simulink model "fbuildv0p3"  (R2024b)
settings: Solver=VariableStepAuto  StartTime=0.0  StopTime=10.0  RelTol=1e-3
model workspace (MAT data in the model file):
  DGain = [16.29965735 16.29965735 15.46224499 15.46224499 15.85491435 21.71073697 22.54158281 11.7271646 11.89023926 12.01707508 12.11854371 12.20156349 12.27074664 12.32928621 12.37946299]
  FBgain = 1
  FFgain = 1
  GR = 14.14
  IGain = [117.4799242 117.4799242 87.54143949 87.54143949 65.86609231 58.19090765 57.39102046 195.6414284 195.4270634 195.2603347 195.1269515 195.0178196 194.9268763 194.8499242 194.7839652]
  Izz = 80
  Kb = 5
  Kd = 2
  Ki = 10
  Kn = 1
  Kp = 0.1
  L = 1.53
  Mz_to_CMD_TV_delta = 1
  NGain = [2.84450804 2.84450804 4.245826716 5.412937893 3.440885499 2 2 14.58729627 14.58729627 14.58729627 14.58729627 14.58729627 14.58729627 14.58729627 14.58729627]
  PGain = [130.03354 130.03354 132.2979663 135.8088906 130.4448578 122.5111241 121.680406 275.8117795 275.6454267 275.5160406 275.4125314 275.3278419 275.2572671 275.1975499 275.1463636]
  R_e = 0.197
  Tmax = 21
  g = 9.81
  h = 0.225
  kappa_desired = 0.2
  mu = 1
  steering_ratio = 1.17517328292
  t = 1.2
  vx_vector = [0 3.21428571429 6.42857142857 9.64285714286 12.8571428571 16.0714285714 19.2857142857 22.5 25.7142857143 28.9285714286 32.1428571429 35.3571428571 38.5714285714 41.7857142857 45]
libraries: slpidlib x2, simulink x1
settings Model: Creator=kara.28  LastModifiedBy=kara.28

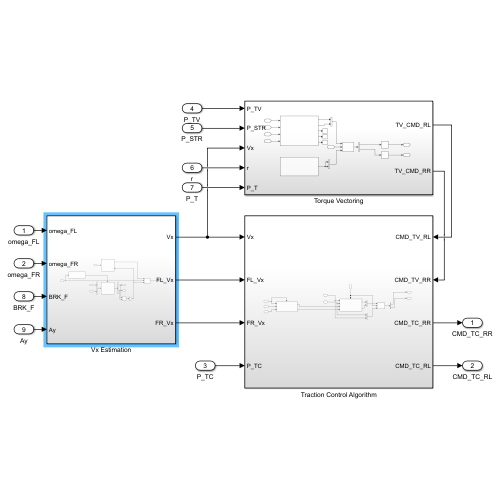
[thumbnail: Simulink's stored preview of the top-level diagram]
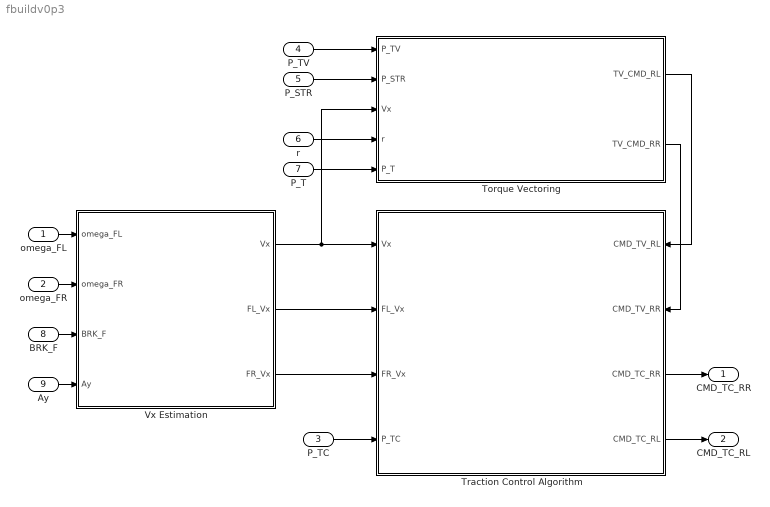
== system fbuildv0p3 ==
  omega_FL : Inport
  omega_FR : Inport  Port=2
  P_TC : Inport  Port=3
  P_TV : Inport  Port=4
  P_STR : Inport  Port=5
  r : Inport  Port=6
  P_T : Inport  Port=7
  BRK_F : Inport  Port=8
  Ay : Inport  Port=9
  Torque Vectoring : Subsystem
  Traction Control Algorithm : Subsystem
      settings: PortSchema="{\"entries\":[{\"content\":{\"sides\":[{\"content\":{\"connectorIds\":[\"In1\",\"In2\",\"In3\",\"In4\"]},\"type\":\"ConnectorPlacement.EquallySpacedRectSide\",\"uuid\":\"6d3224cc-3493-4876-87bf-cb750c54d205\"},{\"content\":{\"connectorIds\":[\"In5\",\"In6\",\"Out1\",\"Out2\"],\"side\":\"RIGHT\"},\"type\":\"ConnectorPlacement.EquallySpacedRectSide\",\"uuid\":\"16bb671c-e18d-4977-8b66-2f7bbb636356\"},{\"content\":{\"side\":\"TOP\"},\"type\":\"ConnectorPlacement.EquallySpacedRectSide\",\"uuid\":\"70c91239-ad82-48f3-8aa3-48d7bdfb7bbb\"}]},\"type\":\"ConnectorPlacement.EquallySpacedConnector\",\"uuid\":\"0f8ba5f7-72f2-430e-8458-63f00911aa7a\"}],\"packageUris\":[\"http://schema.mathworks.com/mf0/Connector/R2020b\"],\"version\":\"1.0\"}"
  Vx Estimation : Subsystem
  CMD_TC_RR : Outport
  CMD_TC_RL : Outport  Port=2
  wires:
  Traction Control Algorithm/2(CMD_TC_RL) -> CMD_TC_RL/1
  Traction Control Algorithm/1(CMD_TC_RR) -> CMD_TC_RR/1
  P_TC/1 -> Traction Control Algorithm/4(P_TC)
  Torque Vectoring/1(TV_CMD_RL) -> Traction Control Algorithm/5(CMD_TV_RL)
  Torque Vectoring/2(TV_CMD_RR) -> Traction Control Algorithm/6(CMD_TV_RR)
  P_TV/1 -> Torque Vectoring/1(P_TV)
  r/1 -> Torque Vectoring/4(r)
  P_T/1 -> Torque Vectoring/5(P_T)
  P_STR/1 -> Torque Vectoring/2(P_STR)
  omega_FL/1 -> Vx Estimation/1(omega_FL)
  omega_FR/1 -> Vx Estimation/2(omega_FR)
  Vx Estimation/2(FL_Vx) -> Traction Control Algorithm/2(FL_Vx)
  Vx Estimation/3(FR_Vx) -> Traction Control Algorithm/3(FR_Vx)
  BRK_F/1 -> Vx Estimation/3(BRK_F)
  Ay/1 -> Vx Estimation/4(Ay)
  Vx Estimation/1(Vx) -> Torque Vectoring/3(Vx), Traction Control Algorithm/1(Vx)

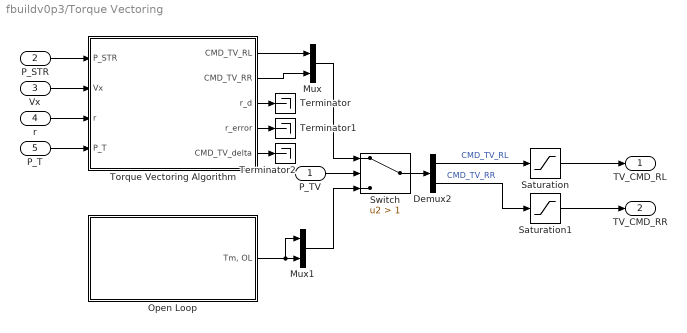
== system fbuildv0p3/Torque Vectoring ==
  P_TV : Inport
  P_STR : Inport  Port=2
  Vx : Inport  Port=3
  r : Inport  Port=4
  P_T : Inport  Port=5
  Demux2 : Demux  Outputs=2
  Mux : Mux  Inputs=2
  Mux1 : Mux  Inputs=2
  Open Loop : Subsystem
  Saturation : Saturate  UpperLimit=Tmax  LowerLimit=0
  Saturation1 : Saturate  UpperLimit=Tmax  LowerLimit=0
  Switch : Switch  Criteria=u2 > Threshold  Threshold=1  SaturateOnIntegerOverflow=off  InputSameDT=off
  Terminator : Terminator
  Terminator1 : Terminator
  Terminator2 : Terminator
  Torque Vectoring Algorithm : Subsystem
  TV_CMD_RL : Outport
  TV_CMD_RR : Outport  Port=2
  wires:
  Demux2/2 -> Saturation1/1  "CMD_TV_RR"
  Mux/1 -> Switch/1
  P_TV/1 -> Switch/2
  Torque Vectoring Algorithm/2(CMD_TV_RR) -> Mux/2
  Demux2/1 -> Saturation/1  "CMD_TV_RL"
  Open Loop/1("Tm, OL") -> Mux1/1, Mux1/2
  Torque Vectoring Algorithm/1(CMD_TV_RL) -> Mux/1
  Mux1/1 -> Switch/3
  Switch/1 -> Demux2/1
  Saturation/1 -> TV_CMD_RL/1
  Saturation1/1 -> TV_CMD_RR/1
  P_STR/1 -> Torque Vectoring Algorithm/1(P_STR)
  Vx/1 -> Torque Vectoring Algorithm/2(Vx)
  r/1 -> Torque Vectoring Algorithm/3(r)
  P_T/1 -> Torque Vectoring Algorithm/4(P_T)
  Torque Vectoring Algorithm/3(r_d) -> Terminator/1
  Torque Vectoring Algorithm/4(r_error) -> Terminator1/1
  Torque Vectoring Algorithm/5(CMD_TV_delta) -> Terminator2/1

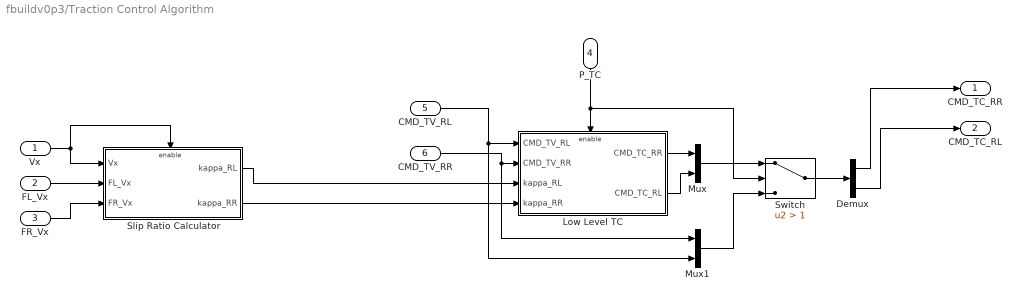
== system fbuildv0p3/Traction Control Algorithm ==
  Vx : Inport
  FL_Vx : Inport  Port=2
  FR_Vx : Inport  Port=3
  P_TC : Inport  Port=4
  CMD_TV_RL : Inport  Port=5
  CMD_TV_RR : Inport  Port=6
  Demux : Demux  Outputs=2
  Low Level TC : Subsystem
  Mux : Mux  Inputs=2
  Mux1 : Mux  Inputs=2
  Slip Ratio Calculator : Subsystem
  Switch : Switch  Criteria=u2 > Threshold  Threshold=1  SaturateOnIntegerOverflow=off  InputSameDT=off
  CMD_TC_RR : Outport
  CMD_TC_RL : Outport  Port=2
  wires:
  Slip Ratio Calculator/2(kappa_RR) -> Low Level TC/4(kappa_RR)
  Slip Ratio Calculator/1(kappa_RL) -> Low Level TC/3(kappa_RL)
  FL_Vx/1 -> Slip Ratio Calculator/2(FL_Vx)
  Vx/1 -> Slip Ratio Calculator/Enable, Slip Ratio Calculator/1(Vx)
  FR_Vx/1 -> Slip Ratio Calculator/3(FR_Vx)
  CMD_TV_RL/1 -> Mux1/2, Low Level TC/1(CMD_TV_RL)
  CMD_TV_RR/1 -> Mux1/1, Low Level TC/2(CMD_TV_RR)
  Low Level TC/1(CMD_TC_RR) -> Mux/1
  Low Level TC/2(CMD_TC_RL) -> Mux/2
  Mux/1 -> Switch/1
  Mux1/1 -> Switch/3
  Switch/1 -> Demux/1
  Demux/1 -> CMD_TC_RR/1
  Demux/2 -> CMD_TC_RL/1
  P_TC/1 -> Switch/2, Low Level TC/Enable

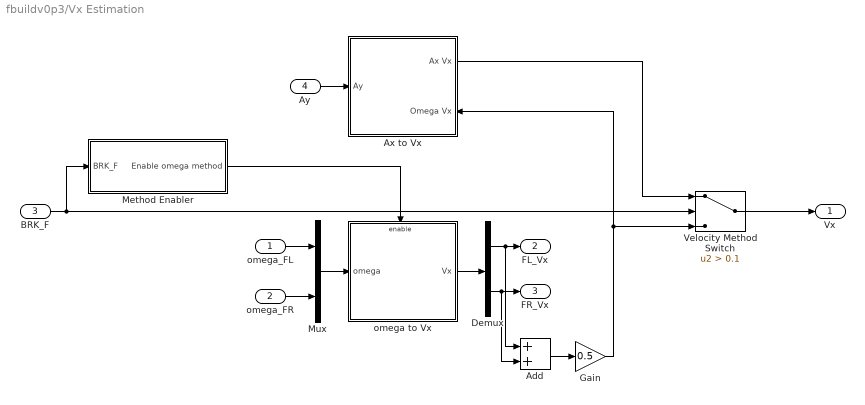
== system fbuildv0p3/Vx Estimation ==
  omega_FL : Inport
  omega_FR : Inport  Port=2
  BRK_F : Inport  Port=3
  Ay : Inport  Port=4
  Add : Sum
  Ax to Vx : Subsystem
      settings: PortSchema="{\"entries\":[{\"content\":{\"sides\":[{\"content\":{\"connectorIds\":[\"In1\"]},\"type\":\"ConnectorPlacement.EquallySpacedRectSide\",\"uuid\":\"79c47d4c-99fc-4629-a356-2be92d656877\"},{\"content\":{\"connectorIds\":[\"Out1\",\"In2\"],\"side\":\"RIGHT\"},\"type\":\"ConnectorPlacement.EquallySpacedRectSide\",\"uuid\":\"a204b3f9-9e82-4b36-9d8a-f01b275c5020\"},{\"content\":{\"side\":\"TOP\"},\"type\":\"ConnectorPlacement.EquallySpacedRectSide\",\"uuid\":\"291354ec-abfe-4550-96ed-63da0986eee3\"}]},\"type\":\"ConnectorPlacement.EquallySpacedConnector\",\"uuid\":\"7bc182f3-54d0-4c5b-b5ad-7c4b2ff36ffe\"}],\"packageUris\":[\"http://schema.mathworks.com/mf0/Connector/R2020b\"],\"version\":\"1.0\"}"
  Demux : Demux  Outputs=2
  Gain : Gain  Gain=0.5
  Method Enabler : Subsystem
  Mux : Mux  Inputs=2
  Velocity Method Switch : Switch  Criteria=u2 > Threshold  Threshold=0.1  SaturateOnIntegerOverflow=off  InputSameDT=off
  omega to Vx : Subsystem
  Vx : Outport
  FL_Vx : Outport  Port=2
  FR_Vx : Outport  Port=3
  wires:
  Mux/1 -> omega to Vx/1(omega)
  omega to Vx/1(Vx) -> Demux/1
  Demux/2 -> Add/2, FR_Vx/1
  omega_FR/1 -> Mux/2
  omega_FL/1 -> Mux/1
  Demux/1 -> Add/1, FL_Vx/1
  BRK_F/1 -> Velocity Method Switch/2, Method Enabler/1(BRK_F)
  Add/1 -> Gain/1
  Gain/1 -> Ax to Vx/2(Omega Vx), Velocity Method Switch/3
  Velocity Method Switch/1 -> Vx/1
  Ay/1 -> Ax to Vx/1(Ay)
  Ax to Vx/1(Ax Vx) -> Velocity Method Switch/1
  Method Enabler/1(Enable omega method) -> omega to Vx/Enable

== system fbuildv0p3/Torque Vectoring/Open Loop ==
  Gain : Gain  Gain=Tmax
  "Tm, OL" : Outport
  wires:
  [throttle] -> Gain/1
  Gain/1 -> "Tm, OL"/1

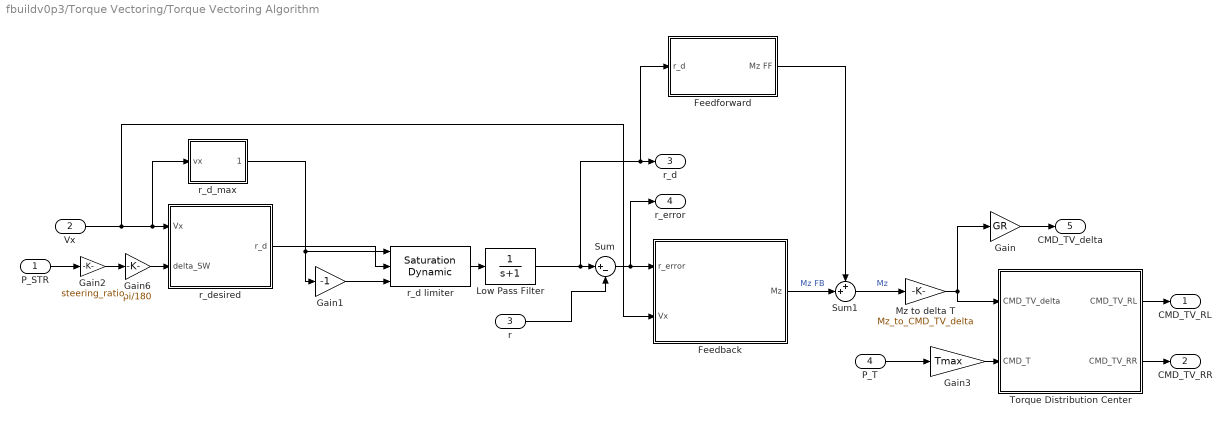
== system fbuildv0p3/Torque Vectoring/Torque Vectoring Algorithm ==
  P_STR : Inport
  Vx : Inport  Port=2
  r : Inport  Port=3
  P_T : Inport  Port=4
  Feedback : Subsystem
  Feedforward : Subsystem
  Gain : Gain  Gain=GR
  Gain1 : Gain  Gain=-1
  Gain2 : Gain  Gain=steering_ratio
  Gain3 : Gain  Gain=Tmax
  Gain6 : Gain  Gain=pi/180
  Low Pass Filter : TransferFcn  Denominator=[1 1]
  Mz to delta T : Gain  Gain=Mz_to_CMD_TV_delta
  Sum : Sum  Inputs=|+-
  Sum1 : Sum  Inputs=++|
  Torque Distribution Center : Subsystem
  r_d limiter : simulink/Discontinuities/Saturation Dynamic  OutMin=[]  OutMax=[]  OutDataTypeStr=Inherit: Same as second input  OutDataType=fixdt(1, 16)  OutScaling=2^-10  RndMeth=Round  DoSatur=off
  r_d_max : Subsystem
  r_desired : Subsystem
  CMD_TV_RL : Outport
  CMD_TV_RR : Outport  Port=2
  r_d : Outport  Port=3
  r_error : Outport  Port=4
  CMD_TV_delta : Outport  Port=5
  wires:
  r_d_max/1(r_d_max) -> r_d limiter/1, Gain1/1
  Sum/1 -> r_error/1, Feedback/1(r_error)
  r_desired/1(r_d) -> r_d limiter/2
  Gain3/1 -> Torque Distribution Center/2(CMD_T)
  r/1 -> Sum/2
  Gain1/1 -> r_d limiter/3
  P_T/1 -> Gain3/1
  Mz to delta T/1 -> Torque Distribution Center/1(CMD_TV_delta), Gain/1
  Gain6/1 -> r_desired/2(delta_SW)
  Vx/1 -> Feedback/2(Vx), r_d_max/1(vx), r_desired/1(Vx)
  Feedback/1(Mz) -> Sum1/2  "Mz FB"
  Sum1/1 -> Mz to delta T/1  "Mz"
  r_d limiter/1 -> Low Pass Filter/1
  Low Pass Filter/1 -> Feedforward/1(r_d), r_d/1, Sum/1
  Feedforward/1(Mz FF) -> Sum1/1
  Torque Distribution Center/1(CMD_TV_RL) -> CMD_TV_RL/1
  Torque Distribution Center/2(CMD_TV_RR) -> CMD_TV_RR/1
  Gain/1 -> CMD_TV_delta/1
  P_STR/1 -> Gain2/1
  Gain2/1 -> Gain6/1

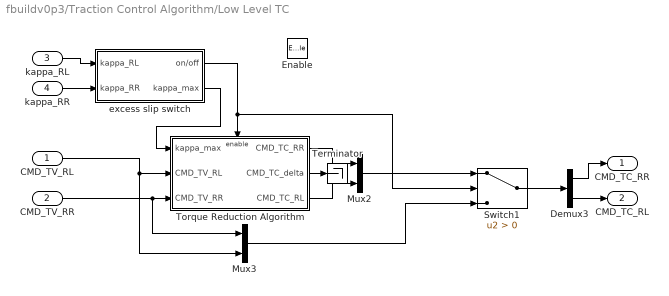
== system fbuildv0p3/Traction Control Algorithm/Low Level TC ==
  CMD_TV_RL : Inport
  CMD_TV_RR : Inport  Port=2
  kappa_RL : Inport  Port=3
  kappa_RR : Inport  Port=4
  Enable : EnablePort
  Demux3 : Demux  Outputs=2
  Mux2 : Mux  Inputs=2
  Mux3 : Mux  Inputs=2
  Switch1 : Switch  Criteria=u2 > Threshold  SaturateOnIntegerOverflow=off  InputSameDT=off
  Terminator : Terminator
  Torque Reduction Algorithm : Subsystem  TreatAsAtomicUnit=on
  excess slip switch : Subsystem
  CMD_TC_RR : Outport
  CMD_TC_RL : Outport  Port=2
  wires:
  Demux3/2 -> CMD_TC_RL/1
  Mux3/1 -> Switch1/3
  CMD_TV_RL/1 -> Mux3/2, Torque Reduction Algorithm/2(CMD_TV_RL)
  Torque Reduction Algorithm/2(CMD_TC_delta) -> Terminator/1
  CMD_TV_RR/1 -> Mux3/1, Torque Reduction Algorithm/3(CMD_TV_RR)
  Torque Reduction Algorithm/1(CMD_TC_RR) -> Mux2/1
  excess slip switch/1(on/off) -> Switch1/2, Torque Reduction Algorithm/Enable
  Mux2/1 -> Switch1/1
  Torque Reduction Algorithm/3(CMD_TC_RL) -> Mux2/2
  Switch1/1 -> Demux3/1
  Demux3/1 -> CMD_TC_RR/1
  excess slip switch/2(kappa_max) -> Torque Reduction Algorithm/1(kappa_max)
  kappa_RL/1 -> excess slip switch/1(kappa_RL)
  kappa_RR/1 -> excess slip switch/2(kappa_RR)

== system fbuildv0p3/Traction Control Algorithm/Slip Ratio Calculator ==
  Vx : Inport
  FL_Vx : Inport  Port=2
  FR_Vx : Inport  Port=3
  Enable : EnablePort
  Divide : Product  Inputs=*/
  Divide1 : Product  Inputs=*/
  Subtract : Sum  Inputs=+-
  Subtract1 : Sum  Inputs=+-
  kappa_RL : Outport
  kappa_RR : Outport  Port=2
  wires:
  Subtract/1 -> Divide/1
  Vx/1 -> Subtract1/1, Divide/2, Divide1/2, Subtract/1
  Divide/1 -> kappa_RL/1
  Divide1/1 -> kappa_RR/1
  Subtract1/1 -> Divide1/1
  FL_Vx/1 -> Subtract/2
  FR_Vx/1 -> Subtract1/2

== system fbuildv0p3/Vx Estimation/Ax to Vx ==
  Ay : Inport
  Omega Vx : Inport  Port=2
  Integrator : Integrator
  Plus : Sum
  Ax Vx : Outport
  wires:
  Ay/1 -> Integrator/1
  Integrator/1 -> Plus/2
  Omega Vx/1 -> Plus/1
  Plus/1 -> Ax Vx/1

== system fbuildv0p3/Vx Estimation/Method Enabler ==
  BRK_F : Inport
  Constant : Constant  Value=0
  Constant1 : Constant
  Switch : Switch  Criteria=u2 > Threshold  Threshold=0.1  SaturateOnIntegerOverflow=off  InputSameDT=off
  Enable omega method : Outport
  wires:
  Constant1/1 -> Switch/3
  Constant/1 -> Switch/1
  Switch/1 -> Enable omega method/1
  BRK_F/1 -> Switch/2

== system fbuildv0p3/Vx Estimation/omega to Vx ==
  omega : Inport
  Enable : EnablePort
  Gain : Gain  Gain=R_e
  Vx : Outport
  wires:
  omega/1 -> Gain/1
  Gain/1 -> Vx/1

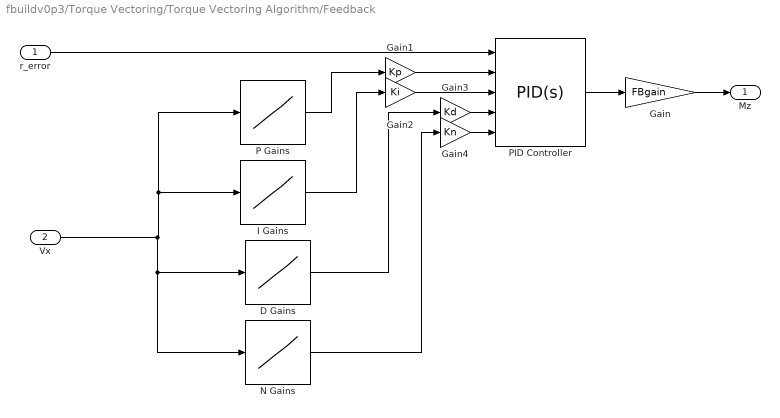
== system fbuildv0p3/Torque Vectoring/Torque Vectoring Algorithm/Feedback ==
  r_error : Inport
  Vx : Inport  Port=2
  D Gains : Lookup_n-D  NumberOfTableDimensions=1  LookupTableObject=''  BreakpointsForDimension1=vx_vector  BreakpointsForDimension1FirstPoint=10  BreakpointsForDimension2FirstPoint=10  BreakpointsForDimension1Spacing=12  BreakpointsForDimension2Spacing=12  IndexSearchMethod=Evenly spaced points  Table=DGain  RemoveProtectionInput=on  InternalRulePriority=Speed  RndMeth=Simplest
  Gain : Gain  Gain=FBgain
  Gain1 : Gain  Gain=Kp
  Gain2 : Gain  Gain=Ki
  Gain3 : Gain  Gain=Kd
  Gain4 : Gain  Gain=Kn
  I Gains : Lookup_n-D  NumberOfTableDimensions=1  LookupTableObject=''  BreakpointsForDimension1=vx_vector  BreakpointsForDimension1FirstPoint=10  BreakpointsForDimension2FirstPoint=10  BreakpointsForDimension1Spacing=12  BreakpointsForDimension2Spacing=12  IndexSearchMethod=Evenly spaced points  Table=IGain  RemoveProtectionInput=on  InternalRulePriority=Speed  RndMeth=Simplest
  N Gains : Lookup_n-D  NumberOfTableDimensions=1  LookupTableObject=''  BreakpointsForDimension1=vx_vector  BreakpointsForDimension1FirstPoint=10  BreakpointsForDimension2FirstPoint=10  BreakpointsForDimension1Spacing=12  BreakpointsForDimension2Spacing=12  IndexSearchMethod=Evenly spaced points  Table=NGain  RemoveProtectionInput=on  InternalRulePriority=Speed  RndMeth=Simplest
  P Gains : Lookup_n-D  NumberOfTableDimensions=1  LookupTableObject=''  BreakpointsForDimension1=vx_vector  BreakpointsForDimension1FirstPoint=10  BreakpointsForDimension2FirstPoint=10  BreakpointsForDimension1Spacing=12  BreakpointsForDimension2Spacing=12  IndexSearchMethod=Evenly spaced points  Table=PGain  RemoveProtectionInput=on  InternalRulePriority=Speed  RndMeth=Simplest
  PID Controller : slpidlib/PID Controller  Controller=PID  Form=Parallel  TimeDomain=Continuous-time  UseExternalTs=off  SampleTime=-1  IntegratorMethod=Forward Euler  FilterMethod=Forward Euler  ControllerParametersSource=external  P=122.511124072632  I=58.1909076470783  UseKiTs=off  D=21.7107369694367  UseExternalDerivativeSource=off  N=2  UseFilter=on  TunerSelectOption=Transfer Function Based (PID Tuner App)  InitialConditionSource=internal  InitialConditionForIntegrator=0  InitialConditionForFilter=0  DifferentiatorICPrevScaledInput=0  ExternalReset=none  TrackingMode=off  Kt=1  LimitOutput=on  SatLimitsSource=internal  UpperSaturationLimit=10  LowerSaturationLimit=-10  LinearizeAsGain=on  AntiWindupMode=back-calculation  Kb=Kb  LimitIntegrator=off  UpperIntegratorSaturationLimit=inf  LowerIntegratorSaturationLimit=-inf  POutMin=[]  POutMax=[]  IOutMin=[]  IOutMax=[]  DOutMin=[]  DOutMax=[]  NOutMin=[]  NOutMax=[]  SumOutMin=[]  SumOutMax=[]  SaturationOutMin=[]  SaturationOutMax=[]  PParamMin=[]  PParamMax=[]  IParamMin=[]  IParamMax=[]  DParamMin=[]  DParamMax=[]  NParamMin=[]  NParamMax=[]  KbParamMin=[]  KbParamMax=[]  KtParamMin=[]  KtParamMax=[]  KbOutMin=[]  KbOutMax=[]  KtOutMin=[]  KtOutMax=[]  IntegratorOutMin=[]  IntegratorOutMax=[]  FilterOutMin=[]  FilterOutMax=[]  SumI1OutMin=[]  SumI1OutMax=[]  SumI2OutMin=[]  SumI2OutMax=[]  SumI3OutMin=[]  SumI3OutMax=[]  SumI4OutMin=[]  SumI4OutMax=[]  SumDOutMin=[]  SumDOutMax=[]  DifferentiatorOutMin=[]  DifferentiatorOutMax=[]  FilterDiffOutCoefMin=[]  FilterDiffOutCoefMax=[]  ReciprocalOutMin=[]  ReciprocalOutMax=[]  SumDenOutMin=[]  SumDenOutMax=[]  SumNumOutMin=[]  SumNumOutMax=[]  DivideOutMin=[]  DivideOutMax=[]  UdiffTsProdOutMin=[]  UdiffTsProdOutMax=[]  NTsProdOutMin=[]  NTsProdOutMax=[]  UintegralTsProdOutMin=[]  UintegralTsProdOutMax=[]  UngainTsProdOutMin=[]  UngainTsProdOutMax=[]  ClampingZeroOutDataTypeStr=Inherit: Inherit via back propagation  ClampingZeroOutMin=[]  ClampingZeroOutMax=[]  FilterDenConstantOutDataTypeStr=Inherit: Inherit via back propagation  FilterDenConstantOutMin=[]  FilterDenConstantOutMax=[]  PCopyOutDataTypeStr=Inherit: Inherit via back propagation  PCopyOutMin=[]  PCopyOutMax=[]  NCopyOutDataTypeStr=Inherit: Inherit via back propagation  NCopyOutMin=[]  NCopyOutMax=[]  IntegratorContinuousStateAttributes=''  IntegratorStateMustResolveToSignalObject=off  IntegratorRTWStateStorageClass=Auto  FilterContinuousStateAttributes=''  FilterStateMustResolveToSignalObject=off  FilterRTWStateStorageClass=Auto  ParallelPVariant=ExternalParameters  IdealPVariant=Disabled  IVariant=ExternalParameters  DVariant=ExternalParameters  IntegratorVariant=Continuous  SatVariant=Enabled  AWVariant=BackCalculation  PCopyVariant=Disabled  TRVariant=Disabled  FdbkBlocksVariant=Forward  IdealPFdbkVariant=Disabled  SatFdbkVariant=Disabled  DerivativeFilterVariant=ContFilter  NVariant=ExternalParameters  NCopyVariant=Disabled  FilterICVariant=InternalICsFilter  IntegratorICVariant=InternalICs  ExternalResetVariant=Disabled  TRSumVariant=Passthrough  SumFdbkVariant=Disabled  SumVariant=Sum_PID  TsampFilterVariant=InternalTs  TsampNgainVariant=Passthrough  TsampIntegralVariant=Disabled_SignalSpec  ExternalSaturationOutDataTypeStr=Inherit: Same as second input  DerivativeSourceVariant=ErrorSignal  PreIntVariant=InternalPreInt
  Mz : Outport
  wires:
  r_error/1 -> PID Controller/1
  Vx/1 -> N Gains/1, D Gains/1, I Gains/1, P Gains/1
  I Gains/1 -> Gain2/1
  N Gains/1 -> Gain4/1
  PID Controller/1 -> Gain/1
  Gain/1 -> Mz/1
  P Gains/1 -> Gain1/1
  D Gains/1 -> Gain3/1
  Gain1/1 -> PID Controller/2
  Gain2/1 -> PID Controller/3
  Gain3/1 -> PID Controller/4
  Gain4/1 -> PID Controller/5

== system fbuildv0p3/Torque Vectoring/Torque Vectoring Algorithm/Feedforward ==
  r_d : Inport
  Gain : Gain  Gain=Izz
  Gain2 : Gain  Gain=FFgain
  Mz FF : Outport
  wires:
  r_d/1 -> Gain/1
  Gain/1 -> Gain2/1
  Gain2/1 -> Mz FF/1  "Mz FF"

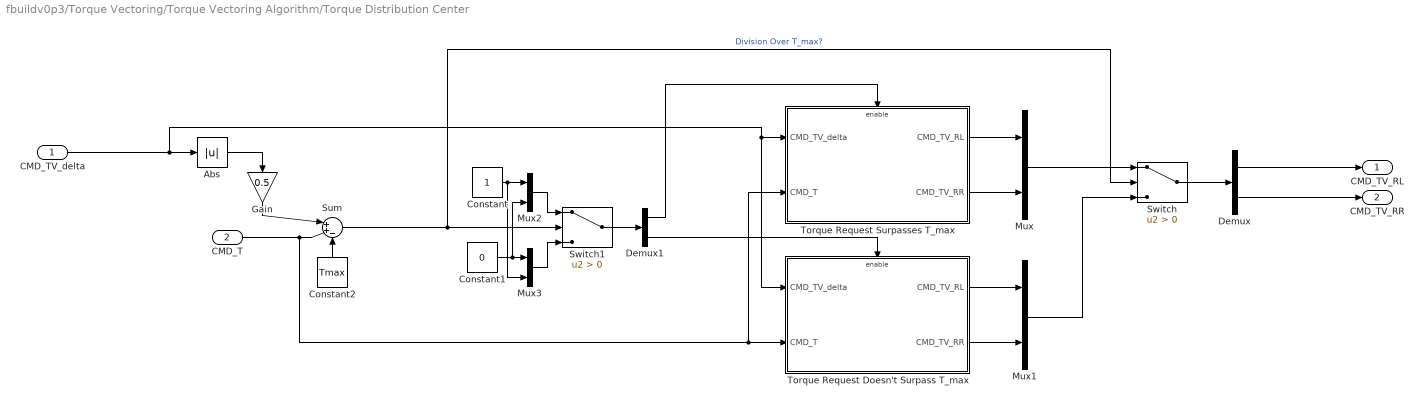
== system fbuildv0p3/Torque Vectoring/Torque Vectoring Algorithm/Torque Distribution Center ==
  CMD_TV_delta : Inport
  CMD_T : Inport  Port=2
  Abs : Abs  SaturateOnIntegerOverflow=off
  Constant : Constant
  Constant1 : Constant  Value=0
  Constant2 : Constant  Value=Tmax
  Demux : Demux  Outputs=2
  Demux1 : Demux  Outputs=2
  Gain : Gain  Gain=0.5
  Mux{,1..3} (4 alike) : Mux  Inputs=2
  Sum : Sum  Inputs=|++-
  Switch : Switch  Criteria=u2 > Threshold  SaturateOnIntegerOverflow=off  InputSameDT=off
  Switch1 : Switch  Criteria=u2 > Threshold  SaturateOnIntegerOverflow=off  InputSameDT=off
  Torque Request Doesn't Surpass T_max : Subsystem  TreatAsAtomicUnit=on
  Torque Request Surpasses T_max : Subsystem  TreatAsAtomicUnit=on
  CMD_TV_RL : Outport
  CMD_TV_RR : Outport  Port=2
  wires:
  Sum/1 -> Switch1/2, Switch/2  "Division Over T_max?"
  Gain/1 -> Sum/1
  Abs/1 -> Gain/1
  Torque Request Surpasses T_max/1(CMD_TV_RL) -> Mux/1
  Torque Request Surpasses T_max/2(CMD_TV_RR) -> Mux/2
  Torque Request Doesn't Surpass T_max/1(CMD_TV_RL) -> Mux1/1
  Torque Request Doesn't Surpass T_max/2(CMD_TV_RR) -> Mux1/2
  Mux/1 -> Switch/1
  Mux1/1 -> Switch/3
  Switch/1 -> Demux/1
  CMD_T/1 -> Torque Request Surpasses T_max/2(CMD_T), Torque Request Doesn't Surpass T_max/2(CMD_T), Sum/2
  Mux2/1 -> Switch1/1
  Mux3/1 -> Switch1/3
  Switch1/1 -> Demux1/1
  Demux1/1 -> Torque Request Surpasses T_max/Enable
  Demux1/2 -> Torque Request Doesn't Surpass T_max/Enable
  Constant/1 -> Mux2/1, Mux3/2
  Constant1/1 -> Mux2/2, Mux3/1
  CMD_TV_delta/1 -> Torque Request Doesn't Surpass T_max/1(CMD_TV_delta), Torque Request Surpasses T_max/1(CMD_TV_delta), Abs/1
  Demux/1 -> CMD_TV_RL/1
  Demux/2 -> CMD_TV_RR/1
  Constant2/1 -> Sum/3

== system fbuildv0p3/Torque Vectoring/Torque Vectoring Algorithm/r_d_max ==
  vx : Inport
  Constant : Constant  Value=0.85*mu*g/(1+(h/t))
  Divide : Product  Inputs=*/
  Saturation : Saturate  UpperLimit=1000000  LowerLimit=0.01
  r_d_max : Outport
  wires:
  Constant/1 -> Divide/1
  vx/1 -> Saturation/1
  Saturation/1 -> Divide/2
  Divide/1 -> r_d_max/1

== system fbuildv0p3/Torque Vectoring/Torque Vectoring Algorithm/r_desired ==
  Vx : Inport
  delta_SW : Inport  Port=2
  Gain : Gain  Gain=1/L
  Product : Product
  Tan : Trigonometry  Operator=tan
  r_d : Outport
  wires:
  delta_SW/1 -> Tan/1
  Vx/1 -> Product/1
  Tan/1 -> Product/2
  Product/1 -> Gain/1
  Gain/1 -> r_d/1

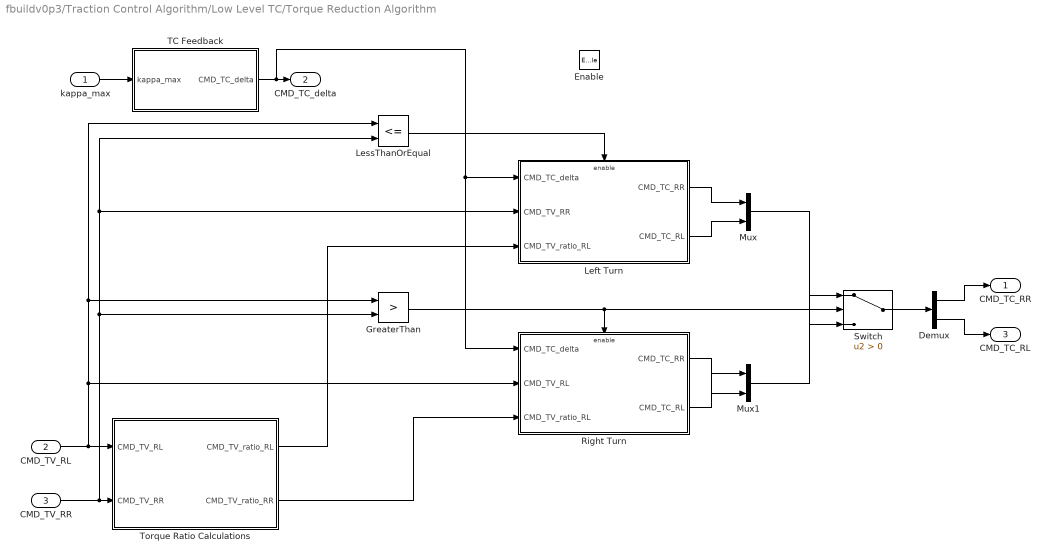
== system fbuildv0p3/Traction Control Algorithm/Low Level TC/Torque Reduction Algorithm ==
  kappa_max : Inport
  CMD_TV_RL : Inport  Port=2
  CMD_TV_RR : Inport  Port=3
  Enable : EnablePort
  Demux : Demux  Outputs=2
  GreaterThan : RelationalOperator  Operator=>  OutDataTypeStr=boolean  RndMeth=Simplest  InputSameDT=off
  Left Turn : Subsystem  TreatAsAtomicUnit=on
  LessThanOrEqual : RelationalOperator  Operator=<=  OutDataTypeStr=boolean  RndMeth=Simplest  InputSameDT=off
  Mux : Mux  Inputs=2
  Mux1 : Mux  Inputs=2
  Right Turn : Subsystem  TreatAsAtomicUnit=on
  Switch : Switch  Criteria=u2 > Threshold  SaturateOnIntegerOverflow=off  InputSameDT=off
  TC Feedback : Subsystem
  Torque Ratio Calculations : Subsystem
  CMD_TC_RR : Outport
  CMD_TC_delta : Outport  Port=2
  CMD_TC_RL : Outport  Port=3
  wires:
  CMD_TV_RL/1 -> GreaterThan/1, LessThanOrEqual/1, Right Turn/2(CMD_TV_RL), Torque Ratio Calculations/1(CMD_TV_RL)
  CMD_TV_RR/1 -> GreaterThan/2, LessThanOrEqual/2, Left Turn/2(CMD_TV_RR), Torque Ratio Calculations/2(CMD_TV_RR)
  LessThanOrEqual/1 -> Left Turn/Enable
  GreaterThan/1 -> Switch/2, Right Turn/Enable
  kappa_max/1 -> TC Feedback/1(kappa_max)
  TC Feedback/1(CMD_TC_delta) -> Right Turn/1(CMD_TC_delta), Left Turn/1(CMD_TC_delta), CMD_TC_delta/1
  Torque Ratio Calculations/1(CMD_TV_ratio_RL) -> Left Turn/3(CMD_TV_ratio_RL)
  Torque Ratio Calculations/2(CMD_TV_ratio_RR) -> Right Turn/3(CMD_TV_ratio_RL)
  Left Turn/1(CMD_TC_RR) -> Mux/1
  Left Turn/2(CMD_TC_RL) -> Mux/2
  Right Turn/2(CMD_TC_RL) -> Mux1/1
  Right Turn/1(CMD_TC_RR) -> Mux1/2
  Mux/1 -> Switch/3
  Mux1/1 -> Switch/1
  Switch/1 -> Demux/1
  Demux/1 -> CMD_TC_RR/1
  Demux/2 -> CMD_TC_RL/1

== system fbuildv0p3/Traction Control Algorithm/Low Level TC/excess slip switch ==
  kappa_RL : Inport
  kappa_RR : Inport  Port=2
  Constant : Constant
  Constant2 : Constant  Value=0
  Max : MinMax  Function=max  Inputs=2
  Switch1 : Switch  Criteria=u2 > Threshold  Threshold=kappa_desired  SaturateOnIntegerOverflow=off  InputSameDT=off
  on/off : Outport
  kappa_max : Outport  Port=2
  wires:
  kappa_RL/1 -> Max/1
  kappa_RR/1 -> Max/2
  Switch1/1 -> on/off/1
  Max/1 -> kappa_max/1, Switch1/2
  Constant2/1 -> Switch1/3
  Constant/1 -> Switch1/1

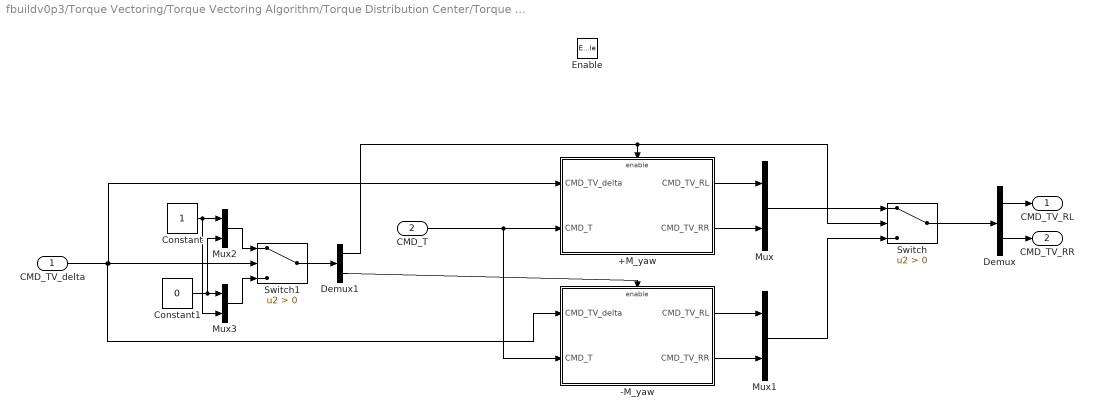
== system fbuildv0p3/Torque Vectoring/Torque Vectoring Algorithm/Torque Distribution Center/Torque Request Doesn't Surpass T_max ==
  CMD_TV_delta : Inport
  CMD_T : Inport  Port=2
  Enable : EnablePort  StatesWhenEnabling=reset
  +M_yaw : Subsystem  TreatAsAtomicUnit=on
  -M_yaw : Subsystem  TreatAsAtomicUnit=on
  Constant : Constant
  Constant1 : Constant  Value=0
  Demux : Demux  Outputs=2
  Demux1 : Demux  Outputs=2
  Mux{,1..3} (4 alike) : Mux  Inputs=2
  Switch : Switch  Criteria=u2 > Threshold  SaturateOnIntegerOverflow=off  InputSameDT=off
  Switch1 : Switch  Criteria=u2 > Threshold  SaturateOnIntegerOverflow=off  InputSameDT=off
  CMD_TV_RL : Outport
  CMD_TV_RR : Outport  Port=2
  wires:
  +M_yaw/1(CMD_TV_RL) -> Mux/1
  +M_yaw/2(CMD_TV_RR) -> Mux/2
  -M_yaw/1(CMD_TV_RL) -> Mux1/1
  -M_yaw/2(CMD_TV_RR) -> Mux1/2
  Mux/1 -> Switch/1
  Mux1/1 -> Switch/3
  CMD_T/1 -> -M_yaw/2(CMD_T), +M_yaw/2(CMD_T)
  Switch/1 -> Demux/1
  Demux/1 -> CMD_TV_RL/1
  Demux/2 -> CMD_TV_RR/1
  Mux2/1 -> Switch1/1
  Demux1/1 -> Switch/2, +M_yaw/Enable
  Demux1/2 -> -M_yaw/Enable
  Mux3/1 -> Switch1/3
  Switch1/1 -> Demux1/1
  Constant1/1 -> Mux2/2, Mux3/1
  Constant/1 -> Mux2/1, Mux3/2
  CMD_TV_delta/1 -> Switch1/2, +M_yaw/1(CMD_TV_delta), -M_yaw/1(CMD_TV_delta)

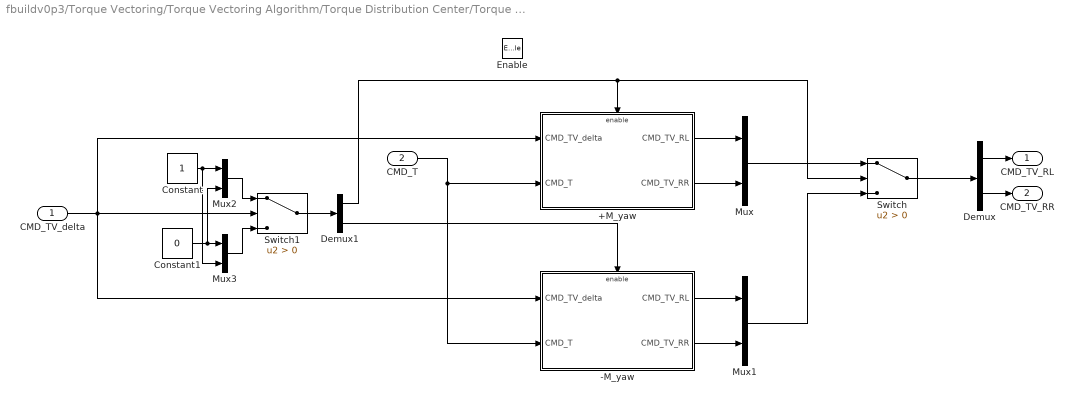
== system fbuildv0p3/Torque Vectoring/Torque Vectoring Algorithm/Torque Distribution Center/Torque Request Surpasses T_max ==
  CMD_TV_delta : Inport
  CMD_T : Inport  Port=2
  Enable : EnablePort  StatesWhenEnabling=reset
  +M_yaw : Subsystem  TreatAsAtomicUnit=on
  -M_yaw : Subsystem  TreatAsAtomicUnit=on
  Constant : Constant
  Constant1 : Constant  Value=0
  Demux : Demux  Outputs=2
  Demux1 : Demux  Outputs=2
  Mux{,1..3} (4 alike) : Mux  Inputs=2
  Switch : Switch  Criteria=u2 > Threshold  SaturateOnIntegerOverflow=off  InputSameDT=off
  Switch1 : Switch  Criteria=u2 > Threshold  SaturateOnIntegerOverflow=off  InputSameDT=off
  CMD_TV_RL : Outport
  CMD_TV_RR : Outport  Port=2
  wires:
  Mux/1 -> Switch/1
  Mux1/1 -> Switch/3
  CMD_T/1 -> -M_yaw/2(CMD_T), +M_yaw/2(CMD_T)
  Demux/2 -> CMD_TV_RR/1
  Demux/1 -> CMD_TV_RL/1
  +M_yaw/2(CMD_TV_RR) -> Mux/2
  +M_yaw/1(CMD_TV_RL) -> Mux/1
  -M_yaw/2(CMD_TV_RR) -> Mux1/2
  Switch/1 -> Demux/1
  -M_yaw/1(CMD_TV_RL) -> Mux1/1
  Mux2/1 -> Switch1/1
  Demux1/1 -> +M_yaw/Enable, Switch/2
  Demux1/2 -> -M_yaw/Enable
  Mux3/1 -> Switch1/3
  Switch1/1 -> Demux1/1
  Constant1/1 -> Mux2/2, Mux3/1
  Constant/1 -> Mux2/1, Mux3/2
  CMD_TV_delta/1 -> Switch1/2, -M_yaw/1(CMD_TV_delta), +M_yaw/1(CMD_TV_delta)

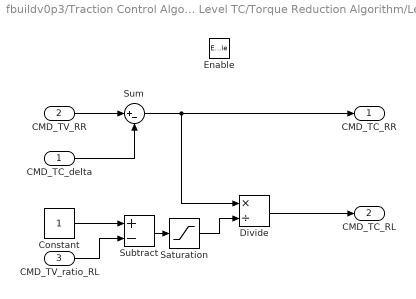
== system fbuildv0p3/Traction Control Algorithm/Low Level TC/Torque Reduction Algorithm/Left Turn ==
  CMD_TC_delta : Inport
  CMD_TV_RR : Inport  Port=2
  CMD_TV_ratio_RL : Inport  Port=3
  Enable : EnablePort
  Constant : Constant
  Divide : Product  Inputs=*/
  Saturation : Saturate  UpperLimit=inf  LowerLimit=0.001
  Subtract : Sum  Inputs=+-
  Sum : Sum  Inputs=|+-
  CMD_TC_RR : Outport
  CMD_TC_RL : Outport  Port=2
  wires:
  CMD_TV_RR/1 -> Sum/1
  CMD_TC_delta/1 -> Sum/2
  Constant/1 -> Subtract/1
  CMD_TV_ratio_RL/1 -> Subtract/2
  Sum/1 -> Divide/1, CMD_TC_RR/1
  Subtract/1 -> Saturation/1
  Saturation/1 -> Divide/2
  Divide/1 -> CMD_TC_RL/1

== system fbuildv0p3/Traction Control Algorithm/Low Level TC/Torque Reduction Algorithm/Right Turn ==
  CMD_TC_delta : Inport
  CMD_TV_RL : Inport  Port=2
  CMD_TV_ratio_RL : Inport  Port=3
  Enable : EnablePort
  Constant : Constant
  Divide : Product  Inputs=*/
  Saturation : Saturate  UpperLimit=inf  LowerLimit=0.001
  Subtract : Sum  Inputs=+-
  Sum : Sum  Inputs=|+-
  CMD_TC_RR : Outport
  CMD_TC_RL : Outport  Port=2
  wires:
  Sum/1 -> Divide/1, CMD_TC_RL/1
  CMD_TC_delta/1 -> Sum/2
  CMD_TV_ratio_RL/1 -> Subtract/2
  Saturation/1 -> Divide/2
  Constant/1 -> Subtract/1
  Subtract/1 -> Saturation/1
  Divide/1 -> CMD_TC_RR/1
  CMD_TV_RL/1 -> Sum/1

== system fbuildv0p3/Traction Control Algorithm/Low Level TC/Torque Reduction Algorithm/TC Feedback ==
  kappa_max : Inport
  Constant : Constant  Value=kappa_desired
  PID Controller : slpidlib/PID Controller  Controller=PID  Form=Parallel  TimeDomain=Continuous-time  UseExternalTs=off  SampleTime=-1  IntegratorMethod=Forward Euler  FilterMethod=Forward Euler  ControllerParametersSource=internal  P=1  I=1  UseKiTs=off  D=0  UseExternalDerivativeSource=off  N=100  UseFilter=on  TunerSelectOption=Transfer Function Based (PID Tuner App)  InitialConditionSource=internal  InitialConditionForIntegrator=0  InitialConditionForFilter=0  DifferentiatorICPrevScaledInput=0  ExternalReset=none  TrackingMode=off  Kt=1  LimitOutput=off  SatLimitsSource=internal  UpperSaturationLimit=inf  LowerSaturationLimit=-inf  LinearizeAsGain=on  AntiWindupMode=none  Kb=1  LimitIntegrator=off  UpperIntegratorSaturationLimit=inf  LowerIntegratorSaturationLimit=-inf  POutMin=[]  POutMax=[]  IOutMin=[]  IOutMax=[]  DOutMin=[]  DOutMax=[]  NOutMin=[]  NOutMax=[]  SumOutMin=[]  SumOutMax=[]  SaturationOutMin=[]  SaturationOutMax=[]  PParamMin=[]  PParamMax=[]  IParamMin=[]  IParamMax=[]  DParamMin=[]  DParamMax=[]  NParamMin=[]  NParamMax=[]  KbParamMin=[]  KbParamMax=[]  KtParamMin=[]  KtParamMax=[]  KbOutMin=[]  KbOutMax=[]  KtOutMin=[]  KtOutMax=[]  IntegratorOutMin=[]  IntegratorOutMax=[]  FilterOutMin=[]  FilterOutMax=[]  SumI1OutMin=[]  SumI1OutMax=[]  SumI2OutMin=[]  SumI2OutMax=[]  SumI3OutMin=[]  SumI3OutMax=[]  SumI4OutMin=[]  SumI4OutMax=[]  SumDOutMin=[]  SumDOutMax=[]  DifferentiatorOutMin=[]  DifferentiatorOutMax=[]  FilterDiffOutCoefMin=[]  FilterDiffOutCoefMax=[]  ReciprocalOutMin=[]  ReciprocalOutMax=[]  SumDenOutMin=[]  SumDenOutMax=[]  SumNumOutMin=[]  SumNumOutMax=[]  DivideOutMin=[]  DivideOutMax=[]  UdiffTsProdOutMin=[]  UdiffTsProdOutMax=[]  NTsProdOutMin=[]  NTsProdOutMax=[]  UintegralTsProdOutMin=[]  UintegralTsProdOutMax=[]  UngainTsProdOutMin=[]  UngainTsProdOutMax=[]  ClampingZeroOutDataTypeStr=Inherit: Inherit via back propagation  ClampingZeroOutMin=[]  ClampingZeroOutMax=[]  FilterDenConstantOutDataTypeStr=Inherit: Inherit via back propagation  FilterDenConstantOutMin=[]  FilterDenConstantOutMax=[]  PCopyOutDataTypeStr=Inherit: Inherit via back propagation  PCopyOutMin=[]  PCopyOutMax=[]  NCopyOutDataTypeStr=Inherit: Inherit via back propagation  NCopyOutMin=[]  NCopyOutMax=[]  IntegratorContinuousStateAttributes=''  IntegratorStateMustResolveToSignalObject=off  IntegratorRTWStateStorageClass=Auto  FilterContinuousStateAttributes=''  FilterStateMustResolveToSignalObject=off  FilterRTWStateStorageClass=Auto  ParallelPVariant=InternalParameters  IdealPVariant=Disabled  IVariant=InternalParameters  DVariant=InternalParameters  IntegratorVariant=Continuous  SatVariant=Disabled  AWVariant=Passthrough  PCopyVariant=Disabled  TRVariant=Disabled  FdbkBlocksVariant=Forward  IdealPFdbkVariant=Disabled  SatFdbkVariant=Disabled  DerivativeFilterVariant=ContFilter  NVariant=InternalParameters  NCopyVariant=Disabled  FilterICVariant=InternalICsFilter  IntegratorICVariant=InternalICs  ExternalResetVariant=Disabled  TRSumVariant=Passthrough  SumFdbkVariant=Disabled  SumVariant=Sum_PID  TsampFilterVariant=InternalTs  TsampNgainVariant=Passthrough  TsampIntegralVariant=Disabled_SignalSpec  ExternalSaturationOutDataTypeStr=Inherit: Same as second input  DerivativeSourceVariant=ErrorSignal  PreIntVariant=InternalPreInt
  Saturation : Saturate  UpperLimit=Tmax  LowerLimit=0
  Sum : Sum  Inputs=|+-
  CMD_TC_delta : Outport
  wires:
  Constant/1 -> Sum/1
  Sum/1 -> PID Controller/1
  PID Controller/1 -> Saturation/1
  kappa_max/1 -> Sum/2
  Saturation/1 -> CMD_TC_delta/1

== system fbuildv0p3/Traction Control Algorithm/Low Level TC/Torque Reduction Algorithm/Torque Ratio Calculations ==
  CMD_TV_RL : Inport
  CMD_TV_RR : Inport  Port=2
  Divide : Product  Inputs=*/
  Divide1 : Product  Inputs=*/
  Saturation : Saturate  UpperLimit=inf  LowerLimit=0.001
  Sum : Sum  Inputs=|++
  CMD_TV_ratio_RL : Outport
  CMD_TV_ratio_RR : Outport  Port=2
  wires:
  CMD_TV_RL/1 -> Divide/1, Sum/1
  CMD_TV_RR/1 -> Sum/2, Divide1/1
  Sum/1 -> Saturation/1
  Saturation/1 -> Divide1/2, Divide/2
  Divide/1 -> CMD_TV_ratio_RL/1
  Divide1/1 -> CMD_TV_ratio_RR/1

== system fbuildv0p3/Torque Vectoring/Torque Vectoring Algorithm/Torque Distribution Center/Torque Request Doesn't Surpass T_max/+M_yaw ==
  CMD_TV_delta : Inport
  CMD_T : Inport  Port=2
  Enable : EnablePort  StatesWhenEnabling=reset
  Abs : Abs  SaturateOnIntegerOverflow=off
  Add : Sum
  Gain : Gain  Gain=0.5
  Subtract : Sum  Inputs=+-
  CMD_TV_RL : Outport
  CMD_TV_RR : Outport  Port=2
  wires:
  CMD_TV_delta/1 -> Abs/1
  Abs/1 -> Gain/1
  Gain/1 -> Add/2, Subtract/2
  CMD_T/1 -> Subtract/1, Add/1
  Subtract/1 -> CMD_TV_RL/1
  Add/1 -> CMD_TV_RR/1

== system fbuildv0p3/Torque Vectoring/Torque Vectoring Algorithm/Torque Distribution Center/Torque Request Doesn't Surpass T_max/-M_yaw ==
  CMD_TV_delta : Inport
  CMD_T : Inport  Port=2
  Enable : EnablePort  StatesWhenEnabling=reset
  Abs : Abs  SaturateOnIntegerOverflow=off
  Add : Sum
  Gain : Gain  Gain=0.5
  Subtract : Sum  Inputs=+-
  CMD_TV_RL : Outport
  CMD_TV_RR : Outport  Port=2
  wires:
  CMD_T/1 -> Subtract/1, Add/1
  Abs/1 -> Gain/1
  Gain/1 -> Add/2, Subtract/2
  CMD_TV_delta/1 -> Abs/1
  Subtract/1 -> CMD_TV_RR/1
  Add/1 -> CMD_TV_RL/1

== system fbuildv0p3/Torque Vectoring/Torque Vectoring Algorithm/Torque Distribution Center/Torque Request Surpasses T_max/+M_yaw ==
  CMD_TV_delta : Inport
  CMD_T : Inport  Port=2
  Enable : EnablePort  StatesWhenEnabling=reset
  Abs : Abs  SaturateOnIntegerOverflow=off
  Constant : Constant  Value=Tmax
  Subtract : Sum  Inputs=+-
  Subtract1 : Sum  Inputs=+-
  Subtract2 : Sum  Inputs=-+
  CMD_TV_RL : Outport
  CMD_TV_RR : Outport  Port=2
  wires:
  Constant/1 -> CMD_TV_RR/1, Subtract/1
  CMD_TV_delta/1 -> Abs/1
  Abs/1 -> Subtract1/1
  CMD_T/1 -> Subtract2/2, Subtract/2
  Subtract/1 -> Subtract1/2
  Subtract1/1 -> Subtract2/1
  Subtract2/1 -> CMD_TV_RL/1

== system fbuildv0p3/Torque Vectoring/Torque Vectoring Algorithm/Torque Distribution Center/Torque Request Surpasses T_max/-M_yaw ==
  CMD_TV_delta : Inport
  CMD_T : Inport  Port=2
  Enable : EnablePort  StatesWhenEnabling=reset
  Abs : Abs  SaturateOnIntegerOverflow=off
  Constant : Constant  Value=Tmax
  Subtract : Sum  Inputs=+-
  Subtract1 : Sum  Inputs=+-
  Subtract2 : Sum  Inputs=-+
  CMD_TV_RL : Outport
  CMD_TV_RR : Outport  Port=2
  wires:
  CMD_T/1 -> Subtract2/2, Subtract/2
  Constant/1 -> CMD_TV_RL/1, Subtract/1
  Subtract/1 -> Subtract1/2
  CMD_TV_delta/1 -> Abs/1
  Subtract1/1 -> Subtract2/1
  Abs/1 -> Subtract1/1
  Subtract2/1 -> CMD_TV_RR/1
